simulink model "Synch_Gen4"  (Simulink 4.00)
settings: Solver=ode23tb  StartTime=0.0  StopTime=5
InitFcn:
  | powericon('psbinitsys',bdroot);
libraries: powerlib_extras x5, powerlib2 x3
settings Model: LastModifiedBy=ieao  SaveTime=off  SaveOutput=off  LimitDataPoints=off  BlockReductionOpt=off

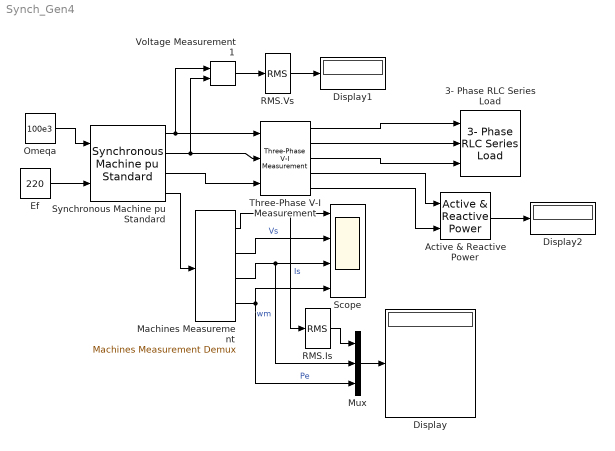
== system Synch_Gen4 ==
  3- Phase RLC Series Load : powerlib_extras/Three-Phase Library/3- Phase RLC Series Load  Vpp=380  fn=50  P3=100e3  QL3=0  QC3=0
  Active & Reactive Power : powerlib_extras/Measurements/Active & Reactive Power  f1=50
  Display : Display
      settings: Format=short  SampleTime=0
  Display1 : Display
      settings: Format=short  SampleTime=0
  Display2 : Display
      settings: Format=short  SampleTime=0
  Ef : Constant  Value=220
  Machines Measurement : powerlib2/Machines/Machines Measurement Demux  machType=Synchronous  ssm1=on  ssm2=on  ssm3=off  ssm4=off  ssm5=on  ssm6=on  sm1=on  sm2=off  sm3=on  sm4=off  sm5=off  sm6=off  sm7=off  sm8=on  sm9=on  sm10=off  sm11=off  asm1=on  asm2=on  asm3=on  asm4=on  asm5=on  asm6=on  asm7=on  asm8=on  asm9=on  asm10=on  asm11=on  pmsm1=on  pmsm2=on  pmsm3=on  pmsm4=on  pmsm5=on  pmsm6=on  lastType=1
  Mux : Mux  Inputs=3
  Omeqa : Constant  Value=100e3
  RMS.Is : powerlib_extras/Measurements/RMS  f1=50
  RMS.Vs : powerlib_extras/Measurements/RMS  f1=50
  Scope : Scope  NumInputPorts=4
      settings: TimeRange=auto  YMin=-7.5~0~0~0  YMax=7.5~70~200~60000  SaveToWorkspace=off  SaveName=ScopeData  MaxDataPoints=5000
  Synchronous Machine pu Standard : powerlib2/Machines/Synchronous Machine pu Standard  Tag=PoWeRsYsTeMbLoCk  rotorType=Salient-pole  x1="[ 187E6  380  50 ]"  x2b=[ 1.81, 0.3, 0.23, 1.76, 0.65, 0.25, 0.15 ]  x2=[ 1.305, 0.296, 0.252, 0.474, 0.243, 0.18 ]  dAxisT=Open-circuit  qAxisT=Short-circuit  x3a="[ 4.4849  0.0681  0.1  ]"  x3b=[ 8.0, 0.03, 1.0, 0.07 ]  x3c="[  4.49  0.0681  0.0513  ]"  x3d=[ 8.0, 0.03, 0.3371, 0.0295 ]  x3=[ 1.01, 0.053, 0.1 ]  x3e=[ 1.3201, 0.023, 1.0, 0.07 ]  x3f="[  1.01  0.053  0.051266  ]"  x3g=[ 1.3201, 0.0231, 0.3371, 0.0295 ]  x4=0.003  x5="[ 3.7 0  20 ]"  x6="[ 0  0  0  0  0  0  0  0  1 ]"  x7=off  x8=[0.6404,0.7127,0.8441,0.9214,0.9956,1.082,1.19,1.316,1.457;0.7,0.7698,0.8872,0.9466,0.9969,1.046,1.1,1.151,1.201]  PSBOutputType=1110  iounits=0.5
  Three-Phase V-I Measurement : powerlib_extras/Measurements/Three-Phase V-I Measurement  phaseurs=off  Vpu=off  Vbase=500e3  Ppu=off  Pbase=100e6
  Voltage Measurement1 : powerlib2/Measurements/Voltage Measurement  Tag=PoWeRsYsTeMmEaSuReMeNt  PSBOutputType=0  PSBequivalent=1
  wires:
  Synchronous Machine pu Standard/1 -> Voltage Measurement1/1, Three-Phase V-I Measurement/1
  Synchronous Machine pu Standard/2 -> Voltage Measurement1/2, Three-Phase V-I Measurement/2
  Synchronous Machine pu Standard/4 -> Machines Measurement/1
  Omeqa/1 -> Synchronous Machine pu Standard/1
  Ef/1 -> Synchronous Machine pu Standard/2
  Machines Measurement/1 -> Scope/1, RMS.Is/1  "Is"
  Voltage Measurement1/1 -> RMS.Vs/1
  RMS.Vs/1 -> Display1/1
  Machines Measurement/2 -> Scope/2  "Vs"
  Machines Measurement/3 -> Scope/3, Mux/2  "wm"
  Machines Measurement/4 -> Scope/4, Mux/3  "Pe"
  RMS.Is/1 -> Mux/1
  Mux/1 -> Display/1
  Synchronous Machine pu Standard/3 -> Three-Phase V-I Measurement/3
  Three-Phase V-I Measurement/4 -> Active & Reactive Power/1
  Three-Phase V-I Measurement/5 -> Active & Reactive Power/2
  Active & Reactive Power/1 -> Display2/1
  Three-Phase V-I Measurement/1 -> 3- Phase RLC Series Load/1
  Three-Phase V-I Measurement/2 -> 3- Phase RLC Series Load/2
  Three-Phase V-I Measurement/3 -> 3- Phase RLC Series Load/3
